simulink model "Project1_part2_opt2_combined"  (R2025b)
settings: Solver=ode45  StartTime=0.0  StopTime=25  FixedStep=1  RelTol=1e-3
values from neighbouring files (symbols this model uses):
  b1 = 1    [run_project1_part2_op3.m]    (also in run_project1_part2_opt1.m; run_project1_part2_opt2.m)
  b2 = 1    [run_project1_part2_op3.m]    (also in run_project1_part2_opt1.m; run_project1_part2_opt2.m)
  J1 = 100    [run_project1_part2_op3.m]    (also in run_project1_part2_opt1.m; run_project1_part2_opt2.m)
  J2 = 1    [run_project1_part2_op3.m]    (also in run_project1_part2_opt1.m; run_project1_part2_opt2.m)
  omega0 = 0    [run_project1_part2_op3.m]    (also in run_project1_part2_opt2.m)
  theta0 = 0    [run_project1_part2_op3.m]    (also in run_project1_part2_opt2.m)
undefined symbols (not defined in the file or in its folder): A
settings Model: Creator=KI5UXW  LastModifiedBy=KI5UXW

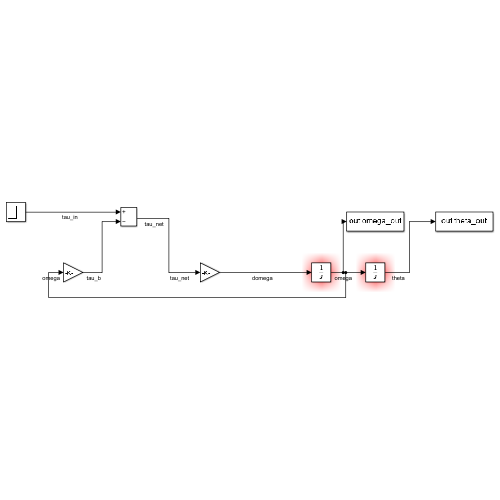
[thumbnail: Simulink's stored preview of the top-level diagram]
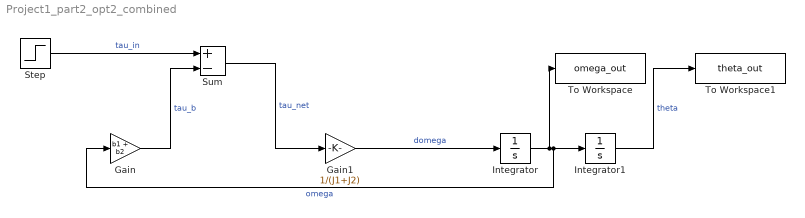
== system Project1_part2_opt2_combined ==
  Gain : Gain  Gain=b1 + b2
  Gain1 : Gain  Gain=1/(J1+J2)
  Integrator : Integrator  InitialCondition=omega0
  Integrator1 : Integrator  InitialCondition=theta0
  Step : Step  Time=0  After=A  SampleTime=0
  Sum : Sum  Inputs=+-
  To Workspace : ToWorkspace  VariableName=omega_out  SaveFormat=Timeseries  SampleTime=-1
  To Workspace1 : ToWorkspace  VariableName=theta_out  SaveFormat=Timeseries  SampleTime=-1
  wires:
  Step/1 -> Sum/1  "tau_in"
  Gain/1 -> Sum/2  "tau_b"
  Gain1/1 -> Integrator/1  "domega"
  Integrator/1 -> To Workspace/1, Gain/1, Integrator1/1  "omega"
  Integrator1/1 -> To Workspace1/1  "theta"
  Sum/1 -> Gain1/1  "tau_net"
